simulink model "w31_v6"  (Simulink 7.9)
settings: Solver=FixedStepDiscrete  StartTime=0.0  StopTime=inf  FixedStep=0.01  RelTol=1e-3
undefined symbols (not defined in the file): DiscIntNeverNeededParam, magnitude
libraries: canmsglib x24, cansrvlib x22, simulink x12, iohwablib x5, legionoslib x3, ccpsrvlib x2, memsrvlib x1, tgttoollib x1, udssrvlib x1, wdgmlib x1
(part 4 of 5)

== system w31_v6/Logic_And_Algorithm/iECU_mode_with_control/Power_calculation/Subsystem ==
  0-1 : Saturate  UpperLimit=1  LowerLimit=0  OutDataTypeStr=uint8
  Constant : Constant  Value=0  OutDataTypeStr=uint8
  Constant1 : Constant  OutDataTypeStr=uint8
  Constant2 : Constant  Value=2  OutDataTypeStr=uint8
  Constant3 : Constant  OutDataTypeStr=uint8
  Constant4 : Constant  Value=0  OutDataTypeStr=uint8
  Constant5 : Constant  OutDataTypeStr=uint8
  Constant6 : Constant  Value=0  OutDataTypeStr=uint8
  Gain : Gain  ParamDataTypeStr=uint8
  Gain1 : Gain  ParamDataTypeStr=uint8
  Multiport Switch : MultiPortSwitch  DataPortOrder=Specify indices  DataPortIndices={0,2,1}  zeroidx=off
  Multiport Switch1 : MultiPortSwitch  DataPortOrder=Specify indices  DataPortIndices={0,1}  zeroidx=off
  Multiport Switch2 : MultiPortSwitch  DataPortOrder=Specify indices  DataPortIndices={0,1}  zeroidx=off
  Rotation_to_FL_Motor : Outport
  Rotation_to_FR_Motor : Outport  Port=2
  Rotation_to_RL_Motor : Outport  Port=3
  Rotation_to_RR_Motor : Outport  Port=4
  tag scope: iECU_GearRequestAfterCal=global
  wires:
  Multiport Switch/1 -> 0-1/1, [iECU_GearRequestAfterCal]  "Rotation_to_RL_Motor"
  Constant/1 -> Multiport Switch/2
  Constant1/1 -> Multiport Switch/3
  Constant2/1 -> Multiport Switch/4
  0-1/1 -> Gain/1, Multiport Switch1/1, Gain1/1, Multiport Switch2/1
  [iECU_GearReq] -> Multiport Switch/1
  Constant3/1 -> Multiport Switch1/2
  Constant4/1 -> Multiport Switch1/3
  Constant5/1 -> Multiport Switch2/2
  Constant6/1 -> Multiport Switch2/3
  Gain/1 -> Rotation_to_FL_Motor/1  "Rotation_to_FL_Motor"
  Multiport Switch1/1 -> Rotation_to_FR_Motor/1  "Rotation_to_FR_Motor"
  Gain1/1 -> Rotation_to_RL_Motor/1  "Rotation_to_RL_Motor"
  Multiport Switch2/1 -> Rotation_to_RR_Motor/1  "Rotation_to_RR_Motor"

== system w31_v6/Logic_And_Algorithm/iECU_mode_with_control/Signal_Input/Emg_No_Msg ==
  note: 急停或信号丢失
  No_iECU_CAN_Msg_Or_Emg_Button : Inport
  Bus Selector3 : BusSelector  OutputSignals=No_iECU_CAN_Msg_Or_Emg_Button
  tag scope: No_iECU_CAN_Msg_Or_Emg_Button=global
  wires:
  Bus Selector3/1 -> [No_iECU_CAN_Msg_Or_Emg_Button]  "<No_iECU_CAN_Msg_Or_Emg_Button>"
  No_iECU_CAN_Msg_Or_Emg_Button/1 -> Bus Selector3/1

== system w31_v6/Logic_And_Algorithm/iECU_mode_with_control/Signal_Input/Hardware_Signal_Goto ==
  Chassis_Receive_input : Inport
  Bus Selector3 : BusSelector  OutputSignals=FL_Motor_Receive.FL_RPM_Feedback,FR_Motor_Receive.FR_RPM_Feedback,RL_Motor_Receive.RL_RPM_Feedback,RR_Motor_Receive.RR_RPM_Feedback
  tag scope: iECU_FL_RPM_Feedback=global, iECU_FR_RPM_Feedback=global, iECU_RL_RPM_Feedback=global, iECU_RR_RPM_Feedback=global
  wires:
  Bus Selector3/3 -> [iECU_RL_RPM_Feedback]  "<RL_RPM_Feedback>"
  Bus Selector3/2 -> [iECU_FR_RPM_Feedback]  "<FR_RPM_Feedback>"
  Bus Selector3/1 -> [iECU_FL_RPM_Feedback]  "<FL_RPM_Feedback>"
  Chassis_Receive_input/1 -> Bus Selector3/1
  Bus Selector3/4 -> [iECU_RR_RPM_Feedback]  "<RR_RPM_Feedback>"

== system w31_v6/Logic_And_Algorithm/iECU_mode_with_control/Signal_Input/Remote_Signal_Goto ==
  Remote_CAN_input : Inport
  Bus Selector3 : BusSelector  OutputSignals=Remote_Analog.Remote_Brake_Pressure_Required
  tag scope: iECU_RemoteBrakePressure=global
  wires:
  Remote_CAN_input/1 -> Bus Selector3/1
  Bus Selector3/1 -> [iECU_RemoteBrakePressure]  "<Remote_Brake_Pressure_Required>"

== system w31_v6/Logic_And_Algorithm/iECU_mode_with_control/Signal_Input/iECU_Signal_Goto ==
  iECU_CAN_input : Inport
  -30~+30 : Saturate  UpperLimit=30  LowerLimit=-30  OutDataTypeStr=Inherit: Inherit via back propagation
  -30~30 : Saturate  UpperLimit=30  LowerLimit=-30  OutDataTypeStr=Inherit: Inherit via back propagation
  Bus Selector3 : BusSelector  OutputSignals=iECU_Speed_Required,iECU_FTire_Angle_Rrquired,iECU_RTire_Angle_Rrquired,iECU_Brake_Pressure_Required,iECU_EPB_Req,iECU_Control_Flag,iECU_Gear_Required,iECU_FTire_Angle_Rrquired,iECU_RTire_Angle_Rrquired,iECU_Status
  tag scope: iECU_BrakePressureReq=global, iECU_Control_Flag=global, iECU_EPB_Req=global, iECU_FTire_Angle_Rrquired=global, iECU_GearReq=global, iECU_RTire_Angle_Rrquired=global, iECU_SpeedLimReq=global, iECU_SpeedReq=global, iECU_Status=global, iECU_SteerModeReq=global
  wires:
  iECU_CAN_input/1 -> Bus Selector3/1
  Bus Selector3/1 -> [iECU_SpeedReq]  "<iECU_Speed_Required>"
  Bus Selector3/2 -> -30~+30/1  "<iECU_FTire_Angle_Rrquired>"
  -30~+30/1 -> [iECU_FTire_Angle_Rrquired]
  Bus Selector3/3 -> -30~30/1  "<iECU_RTire_Angle_Rrquired>"
  -30~30/1 -> [iECU_RTire_Angle_Rrquired]
  Bus Selector3/4 -> [iECU_BrakePressureReq]  "<iECU_Brake_Pressure_Required>"
  Bus Selector3/5 -> [iECU_EPB_Req]  "<iECU_EPB_Req>"
  Bus Selector3/6 -> [iECU_Control_Flag]  "<iECU_Control_Flag>"
  Bus Selector3/7 -> [iECU_GearReq]  "<iECU_Gear_Required>"
  Bus Selector3/8 -> [iECU_SpeedLimReq]  "<iECU_FTire_Angle_Rrquired>"
  Bus Selector3/9 -> [iECU_SteerModeReq]  "<iECU_RTire_Angle_Rrquired>"
  Bus Selector3/10 -> [iECU_Status]  "<iECU_Status>"

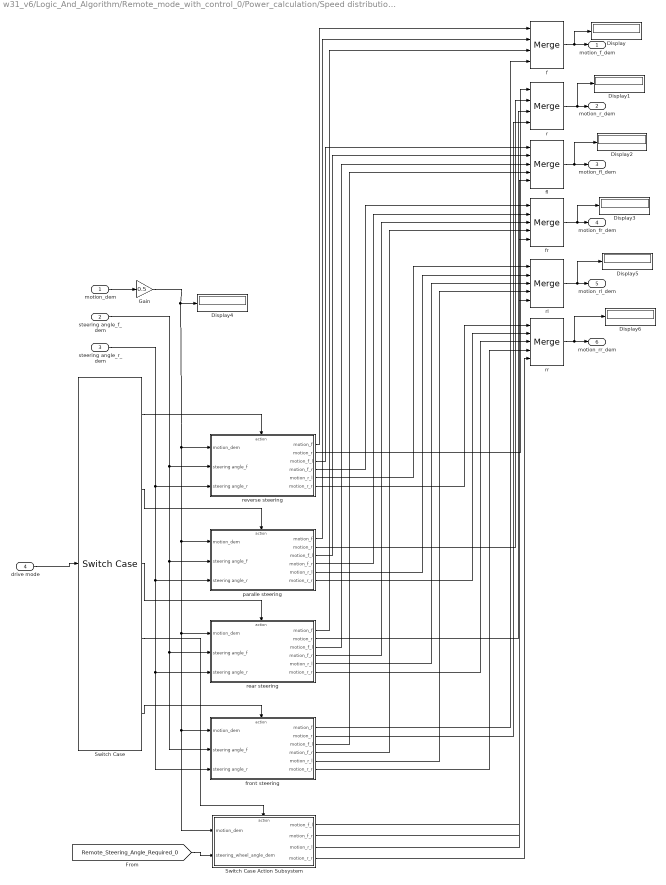
== system w31_v6/Logic_And_Algorithm/Remote_mode_with_control_0/Power_calculation/Speed distribution strategy/motion distribution1 ==
  motion_dem : Inport
  steering angle_f_dem : Inport  Port=2
  steering angle_r_dem : Inport  Port=3
  drive mode : Inport  Port=4
  Display{,1..6} (7 alike) : Display
  Gain : Gain  Gain=0.5
  Switch Case : SwitchCase  CaseConditions={3,0,2,4}
  Switch Case Action Subsystem : Subsystem  TreatAsAtomicUnit=on
  f : Merge  Inputs=4
  fl : Merge  Inputs=5
  fr : Merge  Inputs=5
  front steering : Subsystem  TreatAsAtomicUnit=on
  paralle steering : Subsystem  TreatAsAtomicUnit=on
  r : Merge  Inputs=4
  rear steering : Subsystem  TreatAsAtomicUnit=on
  reverse steering : Subsystem  TreatAsAtomicUnit=on
  rl : Merge  Inputs=5
  rr : Merge  Inputs=5
  motion_f_dem : Outport
  motion_r_dem : Outport  Port=2
  motion_fl_dem : Outport  Port=3
  motion_fr_dem : Outport  Port=4
  motion_rl_dem : Outport  Port=5
  motion_rr_dem : Outport  Port=6
  wires:
  drive mode/1 -> Switch Case/1
  Switch Case/1 -> reverse steering/Action
  Switch Case/2 -> paralle steering/Action
  Switch Case/5 -> front steering/Action
  Switch Case/3 -> rear steering/Action
  reverse steering/3(motion_f_l) -> fl/1
  reverse steering/4(motion_f_r) -> fr/1
  reverse steering/6(motion_r_r) -> rr/1
  paralle steering/3(motion_f_l) -> fl/2
  rear steering/3(motion_f_l) -> fl/3
  front steering/3(motion_f_l) -> fl/4
  paralle steering/4(motion_f_r) -> fr/2
  rear steering/4(motion_f_r) -> fr/3
  front steering/4(motion_f_r) -> fr/4
  reverse steering/5(motion_r_l) -> rl/1
  paralle steering/5(motion_r_l) -> rl/2
  rear steering/5(motion_r_l) -> rl/3
  front steering/5(motion_r_l) -> rl/4
  paralle steering/6(motion_r_r) -> rr/2
  rear steering/6(motion_r_r) -> rr/3
  front steering/6(motion_r_r) -> rr/4
  rr/1 -> motion_rr_dem/1, Display6/1
  rl/1 -> motion_rl_dem/1, Display5/1
  fr/1 -> motion_fr_dem/1, Display3/1
  fl/1 -> motion_fl_dem/1, Display2/1
  f/1 -> motion_f_dem/1, Display/1
  r/1 -> motion_r_dem/1, Display1/1
  reverse steering/1(motion_f) -> f/1
  paralle steering/1(motion_f) -> f/2
  rear steering/1(motion_f) -> f/3
  front steering/1(motion_f) -> f/4
  reverse steering/2(motion_r) -> r/1
  paralle steering/2(motion_r) -> r/2
  rear steering/2(motion_r) -> r/3
  front steering/2(motion_r) -> r/4
  motion_dem/1 -> Gain/1
  steering angle_f_dem/1 -> paralle steering/2(steering angle_f), rear steering/2(steering angle_f), front steering/2(steering angle_f), reverse steering/2(steering angle_f)
  steering angle_r_dem/1 -> reverse steering/3(steering angle_r), rear steering/3(steering angle_r), front steering/3(steering angle_r), paralle steering/3(steering angle_r)
  Switch Case/4 -> Switch Case Action Subsystem/Action
  Switch Case Action Subsystem/1(motion_f_l) -> fl/5
  Switch Case Action Subsystem/2(motion_f_r) -> fr/5
  Switch Case Action Subsystem/3(motion_r_l) -> rl/5
  Switch Case Action Subsystem/4(motion_r_r) -> rr/5
  [Remote_Steering_Angle_Required_0] -> Switch Case Action Subsystem/2(steering_wheel_angle_dem)
  Gain/1 -> reverse steering/1(motion_dem), rear steering/1(motion_dem), front steering/1(motion_dem), Switch Case Action Subsystem/1(motion_dem), paralle steering/1(motion_dem), Display4/1

== system w31_v6/Logic_And_Algorithm/Remote_mode_with_control_0/Steering_calculation/Angle_Cal/F_Steer_mode ==
  Remote_steering : Inport
  Action Port : ActionPort  ActionType=default
  Gain : Gain  Gain=1.2
  Gain1 : Gain  Gain=0
  F_Steering_Angle : Outport
  R_Steering_Angle : Outport  Port=2
  wires:
  Remote_steering/1 -> Gain/1, Gain1/1  "Remote_Steering_Request"
  Gain/1 -> F_Steering_Angle/1  "F_Steering_Angle"
  Gain1/1 -> R_Steering_Angle/1  "R_Steering_Angle"

== system w31_v6/Logic_And_Algorithm/Remote_mode_with_control_0/Steering_calculation/Angle_Cal/Parallel_Steer_mode ==
  Remote_steering : Inport
  Action Port : ActionPort  ActionType=case
  Gain1 : Gain  Gain=1.2
  Tire2EPS : Gain  Gain=1.2
  F_Steering_Angle : Outport
  R_Steering_Angle : Outport  Port=2
  wires:
  Remote_steering/1 -> Tire2EPS/1, Gain1/1  "Remote_Steering_Request"
  Tire2EPS/1 -> F_Steering_Angle/1  "F_Steering_Angle"
  Gain1/1 -> R_Steering_Angle/1  "R_Steering_Angle"

== system w31_v6/Logic_And_Algorithm/Remote_mode_with_control_0/Steering_calculation/Angle_Cal/R_Steer_mode ==
  Remote_steering : Inport
  Action Port : ActionPort  ActionType=case
  Gain : Gain  Gain=0
  Gain1 : Gain  Gain=1.2
  F_Steering_Angle : Outport
  R_Steering_Angle : Outport  Port=2
  wires:
  Remote_steering/1 -> Gain/1, Gain1/1  "Remote_Steering_Request"
  Gain/1 -> F_Steering_Angle/1  "F_Steering_Angle"
  Gain1/1 -> R_Steering_Angle/1  "R_Steering_Angle"

== system w31_v6/Logic_And_Algorithm/Remote_mode_with_control_0/Steering_calculation/Angle_Cal/Reverse_Steer_mode ==
  Remote_steering : Inport
  Action Port : ActionPort  ActionType=case
  Gain : Gain  Gain=1.2
  Gain1 : Gain  Gain=-1.2
  F_Steering_Angle : Outport
  R_Steering_Angle : Outport  Port=2
  wires:
  Remote_steering/1 -> Gain/1, Gain1/1  "Remote_Steering_Request"
  Gain/1 -> F_Steering_Angle/1  "F_Steering_Angle"
  Gain1/1 -> R_Steering_Angle/1  "R_Steering_Angle"

== system w31_v6/Logic_And_Algorithm/Remote_mode_with_control_0/Steering_calculation/Angle_Cal/Steer_Model_Judge ==
  Data Type Conversion : DataTypeConversion  OutDataTypeStr=double
  Data Type Conversion1 : DataTypeConversion  OutDataTypeStr=double
  Data Type Conversion2 : DataTypeConversion  OutDataTypeStr=uint8
  MATLAB Function : MATLAB Function  TreatAsAtomicUnit=on
  Steering_mode : Outport
  tag scope: steering_mode_0=global
  wires:
  MATLAB Function/1(mode) -> Data Type Conversion2/1
  Data Type Conversion/1 -> MATLAB Function/1(steer_gear)
  Data Type Conversion1/1 -> MATLAB Function/2(D_button)
  Data Type Conversion2/1 -> Steering_mode/1, [steering_mode_0]
  [Remote_Steering_Mode_Switch1_0] -> Data Type Conversion/1
  [Remote_Steering_Mode_Switch2_0] -> Data Type Conversion1/1

== system w31_v6/Logic_And_Algorithm/Remote_mode_with_control_0/Steering_calculation/Angle_Cal/turn_in_place ==
  Remote_steering : Inport
  Action Port : ActionPort  ActionType=case
  Gain : Gain  Gain=0
  Gain1 : Gain  Gain=0
  Gain2 : Gain
  F_Steering_Angle : Outport
  R_Steering_Angle : Outport  Port=2
  wires:
  Remote_steering/1 -> Gain2/1  "Remote_Steering_Request"
  Gain/1 -> F_Steering_Angle/1  "F_Steering_Angle"
  Gain1/1 -> R_Steering_Angle/1  "R_Steering_Angle"
  Gain2/1 -> Gain/1, Gain1/1

== system w31_v6/Logic_And_Algorithm/Remote_mode_with_control_2/Steering_calculation/Angle_Cal/F_Steer_mode ==
  Remote_steering : Inport
  Action Port : ActionPort  ActionType=default
  Gain : Gain
  Gain1 : Gain  Gain=0
  F_Steering_Angle : Outport
  R_Steering_Angle : Outport  Port=2
  wires:
  Gain1/1 -> R_Steering_Angle/1  "R_Steering_Angle"
  Gain/1 -> F_Steering_Angle/1  "F_Steering_Angle"
  Remote_steering/1 -> Gain1/1, Gain/1  "Remote_Steering_Request"

== system w31_v6/Logic_And_Algorithm/Remote_mode_with_control_2/Steering_calculation/Angle_Cal/Parallel_Steer_mode ==
  Remote_steering : Inport
  Action Port : ActionPort  ActionType=case
  Gain1 : Gain
  Tire2EPS : Gain
  F_Steering_Angle : Outport
  R_Steering_Angle : Outport  Port=2
  wires:
  Gain1/1 -> R_Steering_Angle/1  "R_Steering_Angle"
  Tire2EPS/1 -> F_Steering_Angle/1  "F_Steering_Angle"
  Remote_steering/1 -> Gain1/1, Tire2EPS/1  "Remote_Steering_Request"

== system w31_v6/Logic_And_Algorithm/Remote_mode_with_control_2/Steering_calculation/Angle_Cal/R_Steer_mode ==
  Remote_steering : Inport
  Action Port : ActionPort  ActionType=case
  Gain : Gain  Gain=0
  Gain1 : Gain
  F_Steering_Angle : Outport
  R_Steering_Angle : Outport  Port=2
  wires:
  Gain1/1 -> R_Steering_Angle/1  "R_Steering_Angle"
  Gain/1 -> F_Steering_Angle/1  "F_Steering_Angle"
  Remote_steering/1 -> Gain1/1, Gain/1  "Remote_Steering_Request"

== system w31_v6/Logic_And_Algorithm/Remote_mode_with_control_2/Steering_calculation/Angle_Cal/Reverse_Steer_mode ==
  Remote_steering : Inport
  Action Port : ActionPort  ActionType=case
  Gain : Gain
  Gain1 : Gain  Gain=-1
  F_Steering_Angle : Outport
  R_Steering_Angle : Outport  Port=2
  wires:
  Gain1/1 -> R_Steering_Angle/1  "R_Steering_Angle"
  Gain/1 -> F_Steering_Angle/1  "F_Steering_Angle"
  Remote_steering/1 -> Gain1/1, Gain/1  "Remote_Steering_Request"

== system w31_v6/Logic_And_Algorithm/Remote_mode_with_control_2/Steering_calculation/Angle_Cal/Steer_Model_Judge ==
  Data Type Conversion : DataTypeConversion  OutDataTypeStr=double
  Data Type Conversion1 : DataTypeConversion  OutDataTypeStr=double
  Data Type Conversion2 : DataTypeConversion  OutDataTypeStr=uint8
  MATLAB Function : MATLAB Function  TreatAsAtomicUnit=on
  Steering_model : Outport
  tag scope: steering_drive_mode2=global
  wires:
  [Remote_Steering_Mode_Switch2_2] -> Data Type Conversion1/1
  [Remote_Steering_Mode_Switch1_2] -> Data Type Conversion/1
  Data Type Conversion2/1 -> Steering_model/1, [steering_drive_mode2]
  Data Type Conversion1/1 -> MATLAB Function/2(D_button)
  Data Type Conversion/1 -> MATLAB Function/1(steer_gear)
  MATLAB Function/1(mode) -> Data Type Conversion2/1

== system w31_v6/Logic_And_Algorithm/Remote_mode_with_control_2/Steering_calculation/Angle_Cal/turn_in_place ==
  Remote_steering : Inport
  Action Port : ActionPort  ActionType=case
  Gain : Gain  Gain=0
  Gain1 : Gain  Gain=0
  Gain2 : Gain
  F_Steering_Angle : Outport
  R_Steering_Angle : Outport  Port=2
  wires:
  Remote_steering/1 -> Gain2/1  "Remote_Steering_Request"
  Gain/1 -> F_Steering_Angle/1  "F_Steering_Angle"
  Gain1/1 -> R_Steering_Angle/1  "R_Steering_Angle"
  Gain2/1 -> Gain/1, Gain1/1

== system w31_v6/Logic_And_Algorithm/iECU_mode_with_control/Power_calculation/PID_Controller/FL_PI_Cal2 ==
  FL_Motor_Error : Inport
  Constant : Constant
  Constant1 : Constant  Value=1.5
  Constant3 : Constant  Value=0
  Constant4 : Constant  Value=0  SampleTime=-1
  Constant5 : Constant  SampleTime=-1
  PI : Subsystem
  Switch : Switch  Criteria=u2 > Threshold
  Switch1 : Switch  Criteria=u2 > Threshold
  Torque_to_FL_Motor : Outport
  wires:
  Constant5/1 -> Switch1/1
  Constant4/1 -> Switch1/3
  [iECU_PID_Reset] -> Switch1/2
  Switch/1 -> Torque_to_FL_Motor/1
  PI/1(PI_闭环计算扭矩) -> Switch/3
  FL_Motor_Error/1 -> PI/1(Error)
  Constant3/1 -> Switch/1
  [iECU_PID_Reset] -> Switch/2
  Constant1/1 -> PI/4(Pgain)
  Constant/1 -> PI/3(Igain)
  Switch1/1 -> PI/2(PID_Reset)

== system w31_v6/Logic_And_Algorithm/iECU_mode_with_control/Power_calculation/PID_Controller/FR_PI_Cal1 ==
  FR_Motor_Error : Inport
  Constant : Constant
  Constant1 : Constant  Value=1.5
  Constant3 : Constant  Value=0
  Constant4 : Constant  Value=0  SampleTime=-1
  Constant5 : Constant  SampleTime=-1
  PI : Subsystem
  Switch : Switch  Criteria=u2 > Threshold
  Switch1 : Switch  Criteria=u2 > Threshold
  Torque_to_FR_Motor : Outport
  wires:
  Switch1/1 -> PI/2(PID_Reset)
  Constant/1 -> PI/3(Igain)
  Constant1/1 -> PI/4(Pgain)
  [iECU_PID_Reset] -> Switch/2
  Constant3/1 -> Switch/1
  FR_Motor_Error/1 -> PI/1(Error)
  PI/1(PI_闭环计算扭矩) -> Switch/3
  Switch/1 -> Torque_to_FR_Motor/1
  [iECU_PID_Reset] -> Switch1/2
  Constant4/1 -> Switch1/3
  Constant5/1 -> Switch1/1

== system w31_v6/Logic_And_Algorithm/iECU_mode_with_control/Power_calculation/PID_Controller/RL_PI_Cal ==
  RL_Motor_Error : Inport
  Constant : Constant
  Constant1 : Constant  Value=1.5
  Constant2 : Constant  Value=0  SampleTime=-1
  Constant3 : Constant  Value=0
  Constant4 : Constant  SampleTime=-1
  PI : Subsystem
  Switch : Switch  Criteria=u2 > Threshold
  Switch1 : Switch  Criteria=u2 > Threshold
  Torque_to_RL_Motor : Outport
  wires:
  Constant/1 -> PI/3(Igain)
  Constant1/1 -> PI/4(Pgain)
  [iECU_PID_Reset] -> Switch/2
  Constant3/1 -> Switch/1
  PI/1(PI_闭环计算扭矩) -> Switch/3
  Switch/1 -> Torque_to_RL_Motor/1
  RL_Motor_Error/1 -> PI/1(Error)
  [iECU_PID_Reset] -> Switch1/2
  Constant2/1 -> Switch1/3
  Constant4/1 -> Switch1/1
  Switch1/1 -> PI/2(PID_Reset)

== system w31_v6/Logic_And_Algorithm/iECU_mode_with_control/Power_calculation/PID_Controller/RR_PI_Cal ==
  RR_Motor_Error : Inport
  Constant : Constant
  Constant1 : Constant  Value=1.5
  Constant3 : Constant  Value=0
  Constant4 : Constant  Value=0  SampleTime=-1
  Constant5 : Constant  SampleTime=-1
  PI : Subsystem
  Switch : Switch  Criteria=u2 > Threshold
  Switch1 : Switch  Criteria=u2 > Threshold
  Torque_to_RR_Motor : Outport
  wires:
  Switch1/1 -> PI/2(PID_Reset)
  Constant/1 -> PI/3(Igain)
  Constant1/1 -> PI/4(Pgain)
  [iECU_PID_Reset] -> Switch/2
  Constant3/1 -> Switch/1
  RR_Motor_Error/1 -> PI/1(Error)
  PI/1(PI_闭环计算扭矩) -> Switch/3
  Switch/1 -> Torque_to_RR_Motor/1
  [iECU_PID_Reset] -> Switch1/2
  Constant4/1 -> Switch1/3
  Constant5/1 -> Switch1/1

== system w31_v6/Logic_And_Algorithm/Remote_mode_with_control_0/Power_calculation/Speed distribution strategy/motion distribution1/Switch Case Action Subsystem ==
  note: 做一个原地转向的限制，轮速不能高于50RPM
  motion_dem : Inport
  steering_wheel_angle_dem : Inport  Port=2
  Action Port : ActionPort  ActionType=case
  MATLAB Function : MATLAB Function  TreatAsAtomicUnit=on
  Product{,1..3} (4 alike) : Product  RndMeth=Zero
  Saturation : Saturate  UpperLimit=50  LowerLimit=-50
  motion_f_l : Outport
  motion_f_r : Outport  Port=2
  motion_r_l : Outport  Port=3
  motion_r_r : Outport  Port=4
  wires:
  steering_wheel_angle_dem/1 -> MATLAB Function/1(steering_wheel_angle_dem)
  motion_dem/1 -> Saturation/1
  MATLAB Function/1(gain1) -> Product/2
  MATLAB Function/2(gain2) -> Product1/2
  MATLAB Function/3(gain3) -> Product2/2
  MATLAB Function/4(gain4) -> Product3/2
  Product/1 -> motion_f_l/1
  Product1/1 -> motion_f_r/1
  Product2/1 -> motion_r_l/1
  Product3/1 -> motion_r_r/1
  Saturation/1 -> Product/1, Product1/1, Product3/1, Product2/1

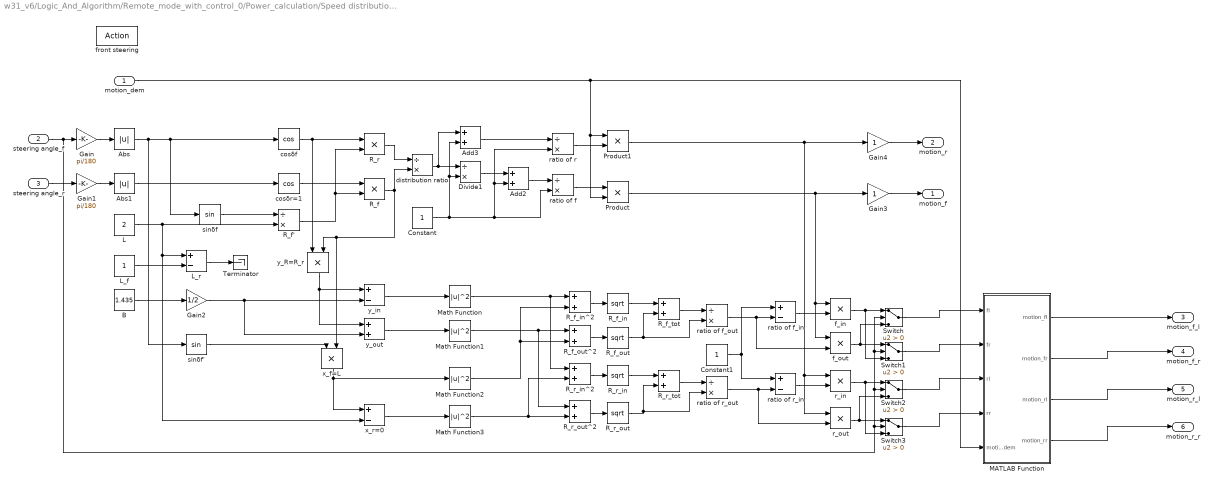
== system w31_v6/Logic_And_Algorithm/Remote_mode_with_control_0/Power_calculation/Speed distribution strategy/motion distribution1/front steering ==
  motion_dem : Inport
  steering angle_f : Inport  Port=2
  steering angle_r : Inport  Port=3
  front steering : ActionPort  ActionType=default
  Abs : Abs
  Abs1 : Abs
  Add2 : Sum
  Add3 : Sum
  B : Constant  Value=1.435
  Constant : Constant
  Constant1 : Constant
  Divide1 : Product  Inputs=/*
  Gain : Gain  Gain=pi/180
  Gain1 : Gain  Gain=pi/180
  Gain2 : Gain  Gain=1/2
  Gain3 : Gain
  Gain4 : Gain
  L : Constant  Value=2
  L_f : Constant
  L_r : Sum  Inputs=+-
  MATLAB Function : MATLAB Function  TreatAsAtomicUnit=on
  Math Function{,1..3} (4 alike) : Math  Operator=magnitude^2  SaturateOnIntegerOverflow=on
  Product : Product
  Product1 : Product
  R_f : Product
  R_f' : Product  Inputs=/*
  R_f_in : Sqrt  SaturateOnIntegerOverflow=on
  R_f_in^2 : Sum
  R_f_out : Sqrt  SaturateOnIntegerOverflow=on
  R_f_out^2 : Sum
  R_f_tot : Sum
  R_r : Product
  R_r_in : Sqrt  SaturateOnIntegerOverflow=on
  R_r_in^2 : Sum
  R_r_out : Sqrt  SaturateOnIntegerOverflow=on
  R_r_out^2 : Sum
  R_r_tot : Sum
  Switch{,1..3} (4 alike) : Switch  Criteria=u2 > Threshold
  Terminator : Terminator
  cosδf : Trigonometry  Operator=cos
  cosδr=1 : Trigonometry  Operator=cos
  distribution ratio : Product  Inputs=/*
  f_in : Product
  f_out : Product
  r_in : Product
  r_out : Product
  ratio of f : Product  Inputs=/*
  ratio of f_in : Sum  Inputs=+-
  ratio of f_out : Product  Inputs=/*
  ratio of r : Product  Inputs=/*
  ratio of r_in : Sum  Inputs=+-
  ratio of r_out : Product  Inputs=/*
  sinδf : Trigonometry
  sinδf' : Trigonometry
  x_f=L : Product
  x_r=0 : Sum  Inputs=+-
  y_R=R_r : Product
  y_in : Sum  Inputs=+-
  y_out : Sum
  motion_f : Outport
  motion_r : Outport  Port=2
  motion_f_l : Outport  Port=3
  motion_f_r : Outport  Port=4
  motion_r_l : Outport  Port=5
  motion_r_r : Outport  Port=6
  wires:
  r_out/1 -> Switch3/1, Switch2/3
  f_out/1 -> Switch1/1, Switch/3
  r_in/1 -> Switch3/3, Switch2/1
  f_in/1 -> Switch/1, Switch1/3
  ratio of f_in/1 -> f_in/2
  ratio of r_in/1 -> r_in/2
  Constant1/1 -> ratio of r_in/1, ratio of f_in/1
  ratio of r_out/1 -> ratio of r_in/2, r_out/2
  ratio of f_out/1 -> ratio of f_in/2, f_out/2
  R_r_tot/1 -> ratio of r_out/1
  R_f_tot/1 -> ratio of f_out/1
  R_r_out/1 -> R_r_tot/2, ratio of r_out/2
  R_r_in/1 -> R_r_tot/1
  R_f_out/1 -> R_f_tot/2, ratio of f_out/2
  R_f_in/1 -> R_f_tot/1
  R_r_out^2/1 -> R_r_out/1
  R_f_out^2/1 -> R_f_out/1
  R_r_in^2/1 -> R_r_in/1
  R_f_in^2/1 -> R_f_in/1
  Math Function3/1 -> R_r_in^2/2, R_r_out^2/2
  Math Function1/1 -> R_f_out^2/1, R_r_out^2/1
  Math Function2/1 -> R_f_in^2/2, R_f_out^2/2
  Math Function/1 -> R_f_in^2/1, R_r_in^2/1
  x_r=0/1 -> Math Function3/1
  y_out/1 -> Math Function1/1
  y_in/1 -> Math Function/1
  x_f=L/1 -> Math Function2/1, x_r=0/1
  L_r/1 -> Terminator/1
  sinδf'/1 -> x_f=L/1
  Gain2/1 -> y_in/2, y_out/2
  y_R=R_r/1 -> y_in/1, y_out/1
  B/1 -> Gain2/1
  Gain1/1 -> Abs1/1
  steering angle_r/1 -> Gain1/1
  Gain/1 -> Abs/1
  steering angle_f/1 -> Gain/1, Switch2/2, Switch/2, Switch1/2, Switch3/2
  Product/1 -> f_out/1, f_in/1, Gain3/1
  Product1/1 -> r_in/1, r_out/1, Gain4/1
  ratio of f/1 -> Product/1
  ratio of r/1 -> Product1/2
  motion_dem/1 -> Product1/1, Product/2, MATLAB Function/5(motion_dem)
  Add3/1 -> ratio of r/1
  Add2/1 -> ratio of f/1
  Divide1/1 -> Add2/1
  Constant/1 -> Divide1/2, Add3/2, Add2/2, ratio of r/2, ratio of f/2
  distribution ratio/1 -> Divide1/1, Add3/1
  R_r/1 -> distribution ratio/1
  R_f/1 -> x_f=L/2, y_R=R_r/2, distribution ratio/2
  R_f'/1 -> R_f/2, R_r/2
  cosδr=1/1 -> R_f/1
  cosδf/1 -> y_R=R_r/1, R_r/1
  sinδf/1 -> R_f'/1
  Abs1/1 -> cosδr=1/1
  Abs/1 -> sinδf/1, cosδf/1, sinδf'/1
  L_f/1 -> L_r/2
  L/1 -> x_r=0/2, L_r/1, R_f'/2
  Gain3/1 -> motion_f/1
  Gain4/1 -> motion_r/1
  Switch/1 -> MATLAB Function/1(fl)
  Switch1/1 -> MATLAB Function/2(fr)
  Switch2/1 -> MATLAB Function/3(rl)
  Switch3/1 -> MATLAB Function/4(rr)
  MATLAB Function/1(motion_fl) -> motion_f_l/1
  MATLAB Function/2(motion_fr) -> motion_f_r/1
  MATLAB Function/3(motion_rl) -> motion_r_l/1
  MATLAB Function/4(motion_rr) -> motion_r_r/1

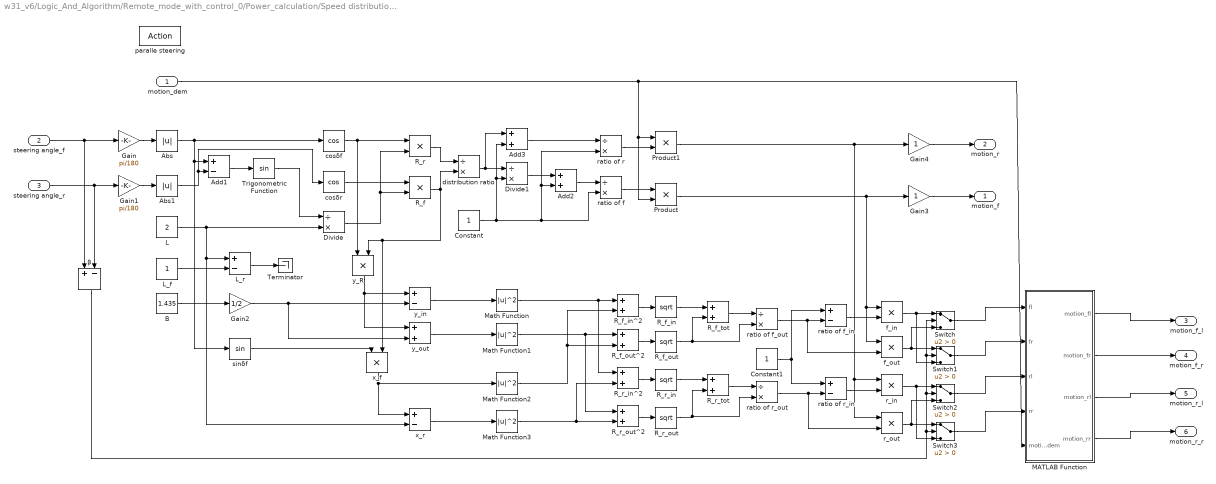
== system w31_v6/Logic_And_Algorithm/Remote_mode_with_control_0/Power_calculation/Speed distribution strategy/motion distribution1/paralle steering ==
  motion_dem : Inport
  steering angle_f : Inport  Port=2
  steering angle_r : Inport  Port=3
  paralle steering : ActionPort  ActionType=case
  Abs : Abs
  Abs1 : Abs
  Add1 : Sum  Inputs=+-
  Add2 : Sum
  Add3 : Sum
  B : Constant  Value=1.435
  Constant : Constant
  Constant1 : Constant
  Divide : Product  Inputs=/*
  Divide1 : Product  Inputs=/*
  Gain : Gain  Gain=pi/180
  Gain1 : Gain  Gain=pi/180
  Gain2 : Gain  Gain=1/2
  Gain3 : Gain
  Gain4 : Gain
  L : Constant  Value=2
  L_f : Constant
  L_r : Sum  Inputs=+-
  MATLAB Function : MATLAB Function  TreatAsAtomicUnit=on
  Math Function{,1..3} (4 alike) : Math  Operator=magnitude^2  SaturateOnIntegerOverflow=on
  Product : Product
  Product1 : Product
  R_f : Product
  R_f_in : Sqrt  SaturateOnIntegerOverflow=on
  R_f_in^2 : Sum
  R_f_out : Sqrt  SaturateOnIntegerOverflow=on
  R_f_out^2 : Sum
  R_f_tot : Sum
  R_r : Product
  R_r_in : Sqrt  SaturateOnIntegerOverflow=on
  R_r_in^2 : Sum
  R_r_out : Sqrt  SaturateOnIntegerOverflow=on
  R_r_out^2 : Sum
  R_r_tot : Sum
  Switch{,1..3} (4 alike) : Switch  Criteria=u2 > Threshold
  Terminator : Terminator
  Trigonometric Function : Trigonometry
  cosδf : Trigonometry  Operator=cos
  cosδr : Trigonometry  Operator=cos
  distribution ratio : Product  Inputs=/*
  f_in : Product
  f_out : Product
  r_in : Product
  r_out : Product
  ratio of f : Product  Inputs=/*
  ratio of f_in : Sum  Inputs=+-
  ratio of f_out : Product  Inputs=/*
  ratio of r : Product  Inputs=/*
  ratio of r_in : Sum  Inputs=+-
  ratio of r_out : Product  Inputs=/*
  sinδf : Trigonometry
  x_f : Product
  x_r : Sum  Inputs=+-
  y_R : Product
  y_in : Sum  Inputs=+-
  y_out : Sum
  β : Sum  Inputs=+-
  motion_f : Outport
  motion_r : Outport  Port=2
  motion_f_l : Outport  Port=3
  motion_f_r : Outport  Port=4
  motion_r_l : Outport  Port=5
  motion_r_r : Outport  Port=6
  wires:
  r_out/1 -> Switch3/1, Switch2/3
  f_out/1 -> Switch1/1, Switch/3
  r_in/1 -> Switch3/3, Switch2/1
  f_in/1 -> Switch/1, Switch1/3
  ratio of f_in/1 -> f_in/2
  ratio of r_in/1 -> r_in/2
  Constant1/1 -> ratio of r_in/1, ratio of f_in/1
  ratio of r_out/1 -> ratio of r_in/2, r_out/2
  ratio of f_out/1 -> ratio of f_in/2, f_out/2
  R_r_tot/1 -> ratio of r_out/1
  R_f_tot/1 -> ratio of f_out/1
  R_r_out/1 -> R_r_tot/2, ratio of r_out/2
  R_r_in/1 -> R_r_tot/1
  R_f_out/1 -> R_f_tot/2, ratio of f_out/2
  R_f_in/1 -> R_f_tot/1
  R_r_out^2/1 -> R_r_out/1
  R_f_out^2/1 -> R_f_out/1
  R_r_in^2/1 -> R_r_in/1
  R_f_in^2/1 -> R_f_in/1
  Math Function3/1 -> R_r_in^2/2, R_r_out^2/2
  Math Function1/1 -> R_f_out^2/1, R_r_out^2/1
  Math Function2/1 -> R_f_in^2/2, R_f_out^2/2
  Math Function/1 -> R_f_in^2/1, R_r_in^2/1
  x_r/1 -> Math Function3/1
  y_out/1 -> Math Function1/1
  y_in/1 -> Math Function/1
  x_f/1 -> Math Function2/1, x_r/1
  L_r/1 -> Terminator/1
  sinδf/1 -> x_f/1
  Gain2/1 -> y_in/2, y_out/2
  y_R/1 -> y_in/1, y_out/1
  B/1 -> Gain2/1
  Gain1/1 -> Abs1/1
  steering angle_r/1 -> Gain1/1, β/2
  Gain/1 -> Abs/1
  β/1 -> Switch2/2, Switch/2, Switch1/2, Switch3/2
  Product/1 -> f_out/1, f_in/1, Gain3/1
  Product1/1 -> r_in/1, r_out/1, Gain4/1
  ratio of f/1 -> Product/1
  ratio of r/1 -> Product1/2
  motion_dem/1 -> Product1/1, Product/2, MATLAB Function/5(motion_dem)
  Add3/1 -> ratio of r/1
  Add2/1 -> ratio of f/1
  Divide1/1 -> Add2/1
  Constant/1 -> Divide1/2, Add3/2, Add2/2, ratio of r/2, ratio of f/2
  distribution ratio/1 -> Divide1/1, Add3/1
  R_r/1 -> distribution ratio/1
  R_f/1 -> distribution ratio/2, x_f/2, y_R/2
  Divide/1 -> R_r/2, R_f/2
  cosδr/1 -> R_f/1
  cosδf/1 -> y_R/1, R_r/1
  Trigonometric Function/1 -> Divide/1
  Add1/1 -> Trigonometric Function/1
  Abs1/1 -> Add1/2, cosδr/1
  Abs/1 -> cosδf/1, Add1/1, sinδf/1
  L_f/1 -> L_r/2
  L/1 -> x_r/2, L_r/1, Divide/2
  steering angle_f/1 -> β/1, Gain/1
  Gain3/1 -> motion_f/1
  Gain4/1 -> motion_r/1
  Switch/1 -> MATLAB Function/1(fl)
  Switch1/1 -> MATLAB Function/2(fr)
  Switch2/1 -> MATLAB Function/3(rl)
  Switch3/1 -> MATLAB Function/4(rr)
  MATLAB Function/1(motion_fl) -> motion_f_l/1
  MATLAB Function/2(motion_fr) -> motion_f_r/1
  MATLAB Function/3(motion_rl) -> motion_r_l/1
  MATLAB Function/4(motion_rr) -> motion_r_r/1

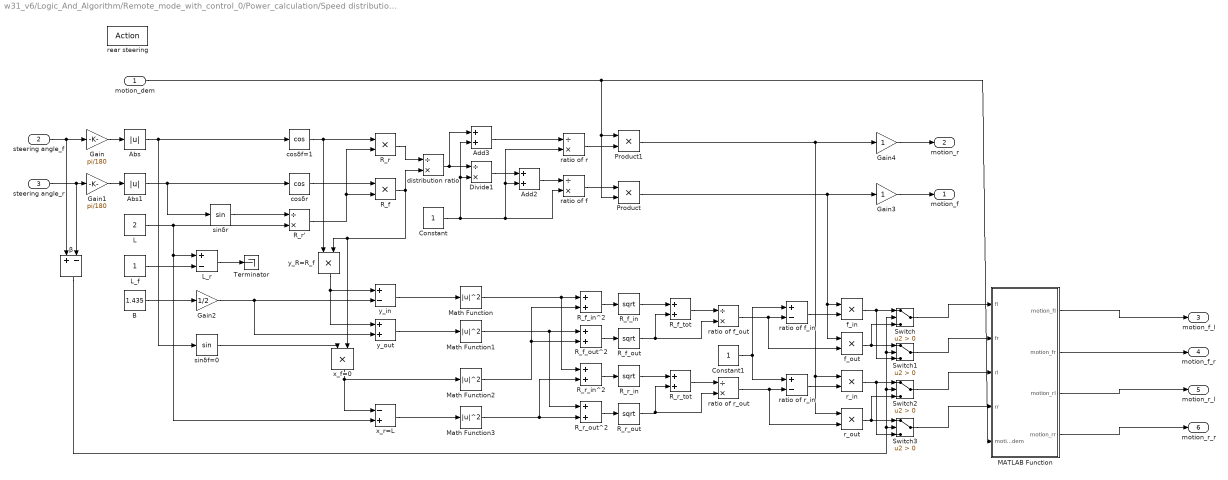
== system w31_v6/Logic_And_Algorithm/Remote_mode_with_control_0/Power_calculation/Speed distribution strategy/motion distribution1/rear steering ==
  motion_dem : Inport
  steering angle_f : Inport  Port=2
  steering angle_r : Inport  Port=3
  rear steering : ActionPort  ActionType=case
  Abs : Abs
  Abs1 : Abs
  Add2 : Sum
  Add3 : Sum
  B : Constant  Value=1.435
  Constant : Constant
  Constant1 : Constant
  Divide1 : Product  Inputs=/*
  Gain : Gain  Gain=pi/180
  Gain1 : Gain  Gain=pi/180
  Gain2 : Gain  Gain=1/2
  Gain3 : Gain
  Gain4 : Gain
  L : Constant  Value=2
  L_f : Constant
  L_r : Sum  Inputs=+-
  MATLAB Function : MATLAB Function  TreatAsAtomicUnit=on
  Math Function{,1..3} (4 alike) : Math  Operator=magnitude^2  SaturateOnIntegerOverflow=on
  Product : Product
  Product1 : Product
  R_f : Product
  R_f_in : Sqrt  SaturateOnIntegerOverflow=on
  R_f_in^2 : Sum
  R_f_out : Sqrt  SaturateOnIntegerOverflow=on
  R_f_out^2 : Sum
  R_f_tot : Sum
  R_r : Product
  R_r' : Product  Inputs=/*
  R_r_in : Sqrt  SaturateOnIntegerOverflow=on
  R_r_in^2 : Sum
  R_r_out : Sqrt  SaturateOnIntegerOverflow=on
  R_r_out^2 : Sum
  R_r_tot : Sum
  Switch{,1..3} (4 alike) : Switch  Criteria=u2 > Threshold
  Terminator : Terminator
  cosδf=1 : Trigonometry  Operator=cos
  cosδr : Trigonometry  Operator=cos
  distribution ratio : Product  Inputs=/*
  f_in : Product
  f_out : Product
  r_in : Product
  r_out : Product
  ratio of f : Product  Inputs=/*
  ratio of f_in : Sum  Inputs=+-
  ratio of f_out : Product  Inputs=/*
  ratio of r : Product  Inputs=/*
  ratio of r_in : Sum  Inputs=+-
  ratio of r_out : Product  Inputs=/*
  sinδf=0 : Trigonometry
  sinδr : Trigonometry
  x_f=0 : Product
  x_r=L : Sum  Inputs=-+
  y_R=R_f : Product
  y_in : Sum  Inputs=+-
  y_out : Sum
  β : Sum  Inputs=+-
  motion_f : Outport
  motion_r : Outport  Port=2
  motion_f_l : Outport  Port=3
  motion_f_r : Outport  Port=4
  motion_r_l : Outport  Port=5
  motion_r_r : Outport  Port=6
  wires:
  L/1 -> R_r'/2, L_r/1, x_r=L/2
  L_f/1 -> L_r/2
  Abs/1 -> sinδf=0/1, cosδf=1/1
  Abs1/1 -> cosδr/1, sinδr/1
  sinδr/1 -> R_r'/1
  cosδf=1/1 -> R_r/1, y_R=R_f/1
  cosδr/1 -> R_f/1
  R_r'/1 -> R_r/2, R_f/2
  R_f/1 -> distribution ratio/2, y_R=R_f/2, x_f=0/2
  R_r/1 -> distribution ratio/1
  distribution ratio/1 -> Add3/1, Divide1/1
  Constant/1 -> ratio of f/2, ratio of r/2, Add2/2, Add3/2, Divide1/2
  Divide1/1 -> Add2/1
  Add2/1 -> ratio of f/1
  Add3/1 -> ratio of r/1
  motion_dem/1 -> Product/2, Product1/1, MATLAB Function/5(motion_dem)
  ratio of r/1 -> Product1/2
  ratio of f/1 -> Product/1
  Product1/1 -> r_out/1, r_in/1, Gain4/1
  Product/1 -> f_in/1, f_out/1, Gain3/1
  β/1 -> Switch3/2, Switch1/2, Switch/2, Switch2/2
  Gain/1 -> Abs/1
  steering angle_r/1 -> β/2, Gain1/1
  Gain1/1 -> Abs1/1
  B/1 -> Gain2/1
  y_R=R_f/1 -> y_out/1, y_in/1
  Gain2/1 -> y_out/2, y_in/2
  sinδf=0/1 -> x_f=0/1
  L_r/1 -> Terminator/1
  x_f=0/1 -> x_r=L/1, Math Function2/1
  y_in/1 -> Math Function/1
  y_out/1 -> Math Function1/1
  x_r=L/1 -> Math Function3/1
  Math Function/1 -> R_r_in^2/1, R_f_in^2/1
  Math Function2/1 -> R_f_out^2/2, R_f_in^2/2
  Math Function1/1 -> R_r_out^2/1, R_f_out^2/1
  Math Function3/1 -> R_r_out^2/2, R_r_in^2/2
  R_f_in^2/1 -> R_f_in/1
  R_r_in^2/1 -> R_r_in/1
  R_f_out^2/1 -> R_f_out/1
  R_r_out^2/1 -> R_r_out/1
  R_f_in/1 -> R_f_tot/1
  R_f_out/1 -> ratio of f_out/2, R_f_tot/2
  R_r_in/1 -> R_r_tot/1
  R_r_out/1 -> ratio of r_out/2, R_r_tot/2
  R_f_tot/1 -> ratio of f_out/1
  R_r_tot/1 -> ratio of r_out/1
  ratio of f_out/1 -> f_out/2, ratio of f_in/2
  ratio of r_out/1 -> r_out/2, ratio of r_in/2
  Constant1/1 -> ratio of f_in/1, ratio of r_in/1
  ratio of r_in/1 -> r_in/2
  ratio of f_in/1 -> f_in/2
  f_in/1 -> Switch1/3, Switch/1
  r_in/1 -> Switch2/1, Switch3/3
  f_out/1 -> Switch/3, Switch1/1
  r_out/1 -> Switch2/3, Switch3/1
  steering angle_f/1 -> Gain/1, β/1
  Gain3/1 -> motion_f/1
  Gain4/1 -> motion_r/1
  Switch/1 -> MATLAB Function/1(fl)
  Switch1/1 -> MATLAB Function/2(fr)
  Switch2/1 -> MATLAB Function/3(rl)
  Switch3/1 -> MATLAB Function/4(rr)
  MATLAB Function/1(motion_fl) -> motion_f_l/1
  MATLAB Function/2(motion_fr) -> motion_f_r/1
  MATLAB Function/3(motion_rl) -> motion_r_l/1
  MATLAB Function/4(motion_rr) -> motion_r_r/1

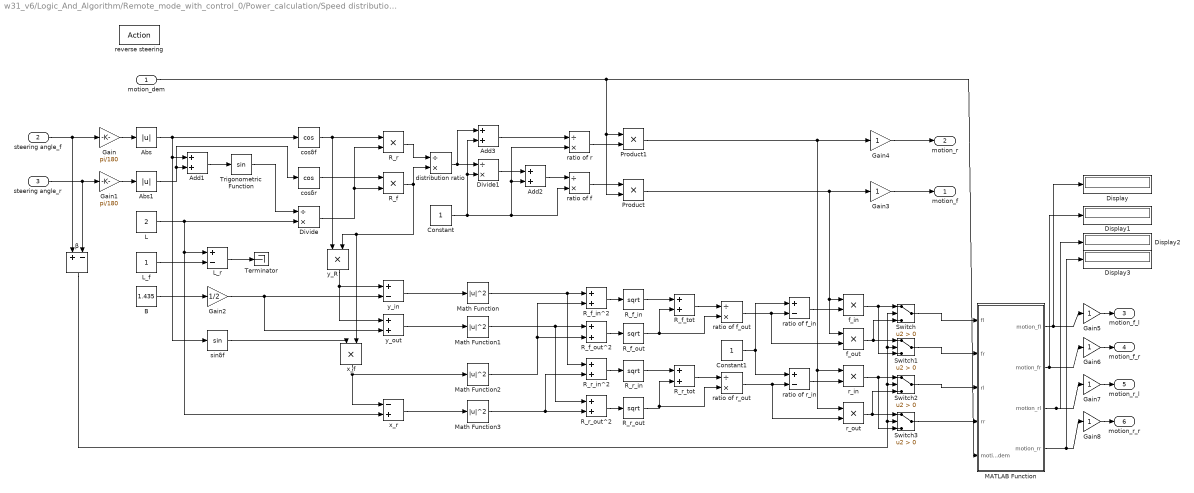
== system w31_v6/Logic_And_Algorithm/Remote_mode_with_control_0/Power_calculation/Speed distribution strategy/motion distribution1/reverse steering ==
  motion_dem : Inport
  steering angle_f : Inport  Port=2
  steering angle_r : Inport  Port=3
  reverse steering : ActionPort  ActionType=case
  Abs : Abs
  Abs1 : Abs
  Add1 : Sum
  Add2 : Sum
  Add3 : Sum
  B : Constant  Value=1.435
  Constant : Constant
  Constant1 : Constant
  Display{,1..3} (4 alike) : Display
  Divide : Product  Inputs=/*
  Divide1 : Product  Inputs=/*
  Gain : Gain  Gain=pi/180
  Gain1 : Gain  Gain=pi/180
  Gain2 : Gain  Gain=1/2
  Gain{3..8} (6 alike) : Gain
  L : Constant  Value=2
  L_f : Constant
  L_r : Sum  Inputs=+-
  MATLAB Function : MATLAB Function  TreatAsAtomicUnit=on
  Math Function{,1..3} (4 alike) : Math  Operator=magnitude^2  SaturateOnIntegerOverflow=on
  Product : Product
  Product1 : Product
  R_f : Product
  R_f_in : Sqrt  SaturateOnIntegerOverflow=on
  R_f_in^2 : Sum
  R_f_out : Sqrt  SaturateOnIntegerOverflow=on
  R_f_out^2 : Sum
  R_f_tot : Sum
  R_r : Product
  R_r_in : Sqrt  SaturateOnIntegerOverflow=on
  R_r_in^2 : Sum
  R_r_out : Sqrt  SaturateOnIntegerOverflow=on
  R_r_out^2 : Sum
  R_r_tot : Sum
  Switch{,1..3} (4 alike) : Switch  Criteria=u2 > Threshold
  Terminator : Terminator
  Trigonometric Function : Trigonometry
  cosδf : Trigonometry  Operator=cos
  cosδr : Trigonometry  Operator=cos
  distribution ratio : Product  Inputs=/*
  f_in : Product
  f_out : Product
  r_in : Product
  r_out : Product
  ratio of f : Product  Inputs=/*
  ratio of f_in : Sum  Inputs=+-
  ratio of f_out : Product  Inputs=/*
  ratio of r : Product  Inputs=/*
  ratio of r_in : Sum  Inputs=+-
  ratio of r_out : Product  Inputs=/*
  sinδf : Trigonometry
  x_f : Product
  x_r : Sum  Inputs=-+
  y_R : Product
  y_in : Sum  Inputs=+-
  y_out : Sum
  β : Sum  Inputs=+-
  motion_f : Outport
  motion_r : Outport  Port=2
  motion_f_l : Outport  Port=3
  motion_f_r : Outport  Port=4
  motion_r_l : Outport  Port=5
  motion_r_r : Outport  Port=6
  wires:
  L/1 -> Divide/2, L_r/1, x_r/2
  L_f/1 -> L_r/2
  Abs/1 -> sinδf/1, Add1/1, cosδf/1
  Abs1/1 -> cosδr/1, Add1/2
  Add1/1 -> Trigonometric Function/1
  Trigonometric Function/1 -> Divide/1
  cosδf/1 -> R_r/1, y_R/1
  cosδr/1 -> R_f/1
  Divide/1 -> R_f/2, R_r/2
  R_f/1 -> y_R/2, x_f/2, distribution ratio/2
  R_r/1 -> distribution ratio/1
  distribution ratio/1 -> Add3/1, Divide1/1
  Constant/1 -> ratio of f/2, ratio of r/2, Add2/2, Add3/2, Divide1/2
  Divide1/1 -> Add2/1
  Add2/1 -> ratio of f/1
  Add3/1 -> ratio of r/1
  motion_dem/1 -> Product/2, Product1/1, MATLAB Function/5(motion_dem)
  ratio of r/1 -> Product1/2
  ratio of f/1 -> Product/1
  Product1/1 -> r_out/1, r_in/1, Gain4/1
  Product/1 -> f_in/1, f_out/1, Gain3/1
  β/1 -> Switch3/2, Switch1/2, Switch/2, Switch2/2
  Gain/1 -> Abs/1
  steering angle_r/1 -> Gain1/1, β/2
  Gain1/1 -> Abs1/1
  B/1 -> Gain2/1
  y_R/1 -> y_out/1, y_in/1
  Gain2/1 -> y_out/2, y_in/2
  sinδf/1 -> x_f/1
  L_r/1 -> Terminator/1
  x_f/1 -> x_r/1, Math Function2/1
  y_in/1 -> Math Function/1
  y_out/1 -> Math Function1/1
  x_r/1 -> Math Function3/1
  Math Function/1 -> R_r_in^2/1, R_f_in^2/1
  Math Function2/1 -> R_f_out^2/2, R_f_in^2/2
  Math Function1/1 -> R_r_out^2/1, R_f_out^2/1
  Math Function3/1 -> R_r_out^2/2, R_r_in^2/2
  R_f_in^2/1 -> R_f_in/1
  R_r_in^2/1 -> R_r_in/1
  R_f_out^2/1 -> R_f_out/1
  R_r_out^2/1 -> R_r_out/1
  R_f_in/1 -> R_f_tot/1
  R_f_out/1 -> ratio of f_out/2, R_f_tot/2
  R_r_in/1 -> R_r_tot/1
  R_r_out/1 -> R_r_tot/2, ratio of r_out/2
  R_f_tot/1 -> ratio of f_out/1
  R_r_tot/1 -> ratio of r_out/1
  ratio of f_out/1 -> f_out/2, ratio of f_in/2
  ratio of r_out/1 -> r_out/2, ratio of r_in/2
  Constant1/1 -> ratio of f_in/1, ratio of r_in/1
  ratio of r_in/1 -> r_in/2
  ratio of f_in/1 -> f_in/2
  f_in/1 -> Switch1/3, Switch/1
  r_in/1 -> Switch2/1, Switch3/3
  f_out/1 -> Switch/3, Switch1/1
  r_out/1 -> Switch2/3, Switch3/1
  steering angle_f/1 -> β/1, Gain/1
  Gain3/1 -> motion_f/1
  Gain4/1 -> motion_r/1
  MATLAB Function/1(motion_fl) -> Gain5/1, Display/1
  MATLAB Function/2(motion_fr) -> Gain6/1, Display1/1
  MATLAB Function/3(motion_rl) -> Gain7/1, Display2/1
  MATLAB Function/4(motion_rr) -> Gain8/1, Display3/1
  Switch/1 -> MATLAB Function/1(fl)
  Switch1/1 -> MATLAB Function/2(fr)
  Switch2/1 -> MATLAB Function/3(rl)
  Switch3/1 -> MATLAB Function/4(rr)
  Gain5/1 -> motion_f_l/1
  Gain6/1 -> motion_f_r/1
  Gain7/1 -> motion_r_l/1
  Gain8/1 -> motion_r_r/1

== system w31_v6/Logic_And_Algorithm/iECU_mode_with_control/Power_calculation/PID_Controller/FL_PI_Cal2/PI ==
  Error : Inport
  PID_Reset : Inport  Port=2
  Igain : Inport  Port=3
  Pgain : Inport  Port=4
  Clamping circuit : Subsystem
  Constant : Constant  Value=0
  Discrete-Time Integrator : DiscreteIntegrator  ExternalReset=level  InitialConditionMode=State only (most efficient)  SampleTime=-1  ICPrevOutput=DiscIntNeverNeededParam  ICPrevScaledInput=DiscIntNeverNeededParam
  Product : Product  RndMeth=Zero
  Product1 : Product  RndMeth=Zero
  Saturation : Saturate  UpperLimit=300  LowerLimit=0
  Sum : Sum  Inputs=++|
  Switch : Switch  Criteria=u2 > Threshold
  PI_闭环计算扭矩 : Outport
  wires:
  Pgain/1 -> Product1/1
  Igain/1 -> Product/2
  Product1/1 -> Sum/1
  PID_Reset/1 -> Discrete-Time Integrator/2
  Saturation/1 -> PI_闭环计算扭矩/1
  Sum/1 -> Clamping circuit/1(preSat), Saturation/1
  Discrete-Time Integrator/1 -> Sum/2
  Switch/1 -> Discrete-Time Integrator/1
  Clamping circuit/1(Clamp) -> Switch/2
  Product/1 -> Clamping circuit/2(preIntegrator), Switch/3
  Constant/1 -> Switch/1
  Error/1 -> Product1/2, Product/1

== system w31_v6/Logic_And_Algorithm/iECU_mode_with_control/Power_calculation/PID_Controller/FR_PI_Cal1/PI ==
  Error : Inport
  PID_Reset : Inport  Port=2
  Igain : Inport  Port=3
  Pgain : Inport  Port=4
  Clamping circuit : Subsystem
  Constant : Constant  Value=0
  Discrete-Time Integrator : DiscreteIntegrator  ExternalReset=level  InitialConditionMode=State only (most efficient)  SampleTime=-1  ICPrevOutput=DiscIntNeverNeededParam  ICPrevScaledInput=DiscIntNeverNeededParam
  Product : Product  RndMeth=Zero
  Product1 : Product  RndMeth=Zero
  Saturation : Saturate  UpperLimit=300  LowerLimit=0
  Sum : Sum  Inputs=++|
  Switch : Switch  Criteria=u2 > Threshold
  PI_闭环计算扭矩 : Outport
  wires:
  Error/1 -> Product/1, Product1/2
  Constant/1 -> Switch/1
  Product/1 -> Switch/3, Clamping circuit/2(preIntegrator)
  Clamping circuit/1(Clamp) -> Switch/2
  Switch/1 -> Discrete-Time Integrator/1
  Discrete-Time Integrator/1 -> Sum/2
  Sum/1 -> Saturation/1, Clamping circuit/1(preSat)
  Saturation/1 -> PI_闭环计算扭矩/1
  PID_Reset/1 -> Discrete-Time Integrator/2
  Product1/1 -> Sum/1
  Igain/1 -> Product/2
  Pgain/1 -> Product1/1

== system w31_v6/Logic_And_Algorithm/iECU_mode_with_control/Power_calculation/PID_Controller/RL_PI_Cal/PI ==
  Error : Inport
  PID_Reset : Inport  Port=2
  Igain : Inport  Port=3
  Pgain : Inport  Port=4
  Clamping circuit : Subsystem
  Constant : Constant  Value=0
  Discrete-Time Integrator : DiscreteIntegrator  ExternalReset=level  InitialConditionMode=State only (most efficient)  SampleTime=-1  ICPrevOutput=DiscIntNeverNeededParam  ICPrevScaledInput=DiscIntNeverNeededParam
  Product : Product  RndMeth=Zero
  Product1 : Product  RndMeth=Zero
  Saturation : Saturate  UpperLimit=300  LowerLimit=0
  Sum : Sum  Inputs=++|
  Switch : Switch  Criteria=u2 > Threshold
  PI_闭环计算扭矩 : Outport
  wires:
  Error/1 -> Product/1, Product1/2
  Constant/1 -> Switch/1
  Product/1 -> Switch/3, Clamping circuit/2(preIntegrator)
  Clamping circuit/1(Clamp) -> Switch/2
  Switch/1 -> Discrete-Time Integrator/1
  Discrete-Time Integrator/1 -> Sum/2
  Sum/1 -> Saturation/1, Clamping circuit/1(preSat)
  Saturation/1 -> PI_闭环计算扭矩/1
  PID_Reset/1 -> Discrete-Time Integrator/2
  Product1/1 -> Sum/1
  Igain/1 -> Product/2
  Pgain/1 -> Product1/1

== system w31_v6/Logic_And_Algorithm/iECU_mode_with_control/Power_calculation/PID_Controller/RR_PI_Cal/PI ==
  Error : Inport
  PID_Reset : Inport  Port=2
  Igain : Inport  Port=3
  Pgain : Inport  Port=4
  Clamping circuit : Subsystem
  Constant : Constant  Value=0
  Discrete-Time Integrator : DiscreteIntegrator  ExternalReset=level  InitialConditionMode=State only (most efficient)  SampleTime=-1  ICPrevOutput=DiscIntNeverNeededParam  ICPrevScaledInput=DiscIntNeverNeededParam
  Product : Product  RndMeth=Zero
  Product1 : Product  RndMeth=Zero
  Saturation : Saturate  UpperLimit=300  LowerLimit=0
  Sum : Sum  Inputs=++|
  Switch : Switch  Criteria=u2 > Threshold
  PI_闭环计算扭矩 : Outport
  wires:
  Error/1 -> Product/1, Product1/2
  Constant/1 -> Switch/1
  Product/1 -> Switch/3, Clamping circuit/2(preIntegrator)
  Clamping circuit/1(Clamp) -> Switch/2
  Switch/1 -> Discrete-Time Integrator/1
  Discrete-Time Integrator/1 -> Sum/2
  Sum/1 -> Saturation/1, Clamping circuit/1(preSat)
  Saturation/1 -> PI_闭环计算扭矩/1
  PID_Reset/1 -> Discrete-Time Integrator/2
  Product1/1 -> Sum/1
  Igain/1 -> Product/2
  Pgain/1 -> Product1/1

== system w31_v6/Logic_And_Algorithm/iECU_mode_with_control/Power_calculation/PID_Controller/FL_PI_Cal2/PI/Clamping circuit ==
  preSat : Inport
  preIntegrator : Inport  Port=2
  Data Type Conversion : DataTypeConversion  OutDataTypeStr=int8  RndMeth=Zero
  Data Type Conversion1 : DataTypeConversion  OutDataTypeStr=int8
  Dead Zone : DeadZone  LowerValue=-250  UpperValue=250
  Logical Operator : Logic  AllPortsSameDT=off  OutDataTypeStr=boolean
  Relational Operator : RelationalOperator  Operator=~=
  Relational Operator1 : RelationalOperator  Operator===
  Sign : Signum
  Sign1 : Signum
  ZeroGain : Gain  Gain=0
  Clamp : Outport
  wires:
  Logical Operator/1 -> Clamp/1
  Relational Operator1/1 -> Logical Operator/2
  Relational Operator/1 -> Logical Operator/1
  Data Type Conversion1/1 -> Relational Operator1/2
  Sign1/1 -> Data Type Conversion1/1
  preIntegrator/1 -> Sign1/1
  Data Type Conversion/1 -> Relational Operator1/1
  Sign/1 -> Data Type Conversion/1
  Dead Zone/1 -> Relational Operator/2, Sign/1
  ZeroGain/1 -> Relational Operator/1
  preSat/1 -> Dead Zone/1, ZeroGain/1

== system w31_v6/Logic_And_Algorithm/iECU_mode_with_control/Power_calculation/PID_Controller/FR_PI_Cal1/PI/Clamping circuit ==
  preSat : Inport
  preIntegrator : Inport  Port=2
  Data Type Conversion : DataTypeConversion  OutDataTypeStr=int8  RndMeth=Zero
  Data Type Conversion1 : DataTypeConversion  OutDataTypeStr=int8
  Dead Zone : DeadZone  LowerValue=-250  UpperValue=250
  Logical Operator : Logic  AllPortsSameDT=off  OutDataTypeStr=boolean
  Relational Operator : RelationalOperator  Operator=~=
  Relational Operator1 : RelationalOperator  Operator===
  Sign : Signum
  Sign1 : Signum
  ZeroGain : Gain  Gain=0
  Clamp : Outport
  wires:
  preSat/1 -> ZeroGain/1, Dead Zone/1
  ZeroGain/1 -> Relational Operator/1
  Dead Zone/1 -> Sign/1, Relational Operator/2
  Sign/1 -> Data Type Conversion/1
  Data Type Conversion/1 -> Relational Operator1/1
  preIntegrator/1 -> Sign1/1
  Sign1/1 -> Data Type Conversion1/1
  Data Type Conversion1/1 -> Relational Operator1/2
  Relational Operator/1 -> Logical Operator/1
  Relational Operator1/1 -> Logical Operator/2
  Logical Operator/1 -> Clamp/1

== system w31_v6/Logic_And_Algorithm/iECU_mode_with_control/Power_calculation/PID_Controller/RL_PI_Cal/PI/Clamping circuit ==
  preSat : Inport
  preIntegrator : Inport  Port=2
  Data Type Conversion : DataTypeConversion  OutDataTypeStr=int8  RndMeth=Zero
  Data Type Conversion1 : DataTypeConversion  OutDataTypeStr=int8
  Dead Zone : DeadZone  LowerValue=-250  UpperValue=250
  Logical Operator : Logic  AllPortsSameDT=off  OutDataTypeStr=boolean
  Relational Operator : RelationalOperator  Operator=~=
  Relational Operator1 : RelationalOperator  Operator===
  Sign : Signum
  Sign1 : Signum
  ZeroGain : Gain  Gain=0
  Clamp : Outport
  wires:
  preSat/1 -> ZeroGain/1, Dead Zone/1
  ZeroGain/1 -> Relational Operator/1
  Dead Zone/1 -> Sign/1, Relational Operator/2
  Sign/1 -> Data Type Conversion/1
  Data Type Conversion/1 -> Relational Operator1/1
  preIntegrator/1 -> Sign1/1
  Sign1/1 -> Data Type Conversion1/1
  Data Type Conversion1/1 -> Relational Operator1/2
  Relational Operator/1 -> Logical Operator/1
  Relational Operator1/1 -> Logical Operator/2
  Logical Operator/1 -> Clamp/1

== system w31_v6/Logic_And_Algorithm/iECU_mode_with_control/Power_calculation/PID_Controller/RR_PI_Cal/PI/Clamping circuit ==
  preSat : Inport
  preIntegrator : Inport  Port=2
  Data Type Conversion : DataTypeConversion  OutDataTypeStr=int8  RndMeth=Zero
  Data Type Conversion1 : DataTypeConversion  OutDataTypeStr=int8
  Dead Zone : DeadZone  LowerValue=-250  UpperValue=250
  Logical Operator : Logic  AllPortsSameDT=off  OutDataTypeStr=boolean
  Relational Operator : RelationalOperator  Operator=~=
  Relational Operator1 : RelationalOperator  Operator===
  Sign : Signum
  Sign1 : Signum
  ZeroGain : Gain  Gain=0
  Clamp : Outport
  wires:
  preSat/1 -> ZeroGain/1, Dead Zone/1
  ZeroGain/1 -> Relational Operator/1
  Dead Zone/1 -> Sign/1, Relational Operator/2
  Sign/1 -> Data Type Conversion/1
  Data Type Conversion/1 -> Relational Operator1/1
  preIntegrator/1 -> Sign1/1
  Sign1/1 -> Data Type Conversion1/1
  Data Type Conversion1/1 -> Relational Operator1/2
  Relational Operator/1 -> Logical Operator/1
  Relational Operator1/1 -> Logical Operator/2
  Logical Operator/1 -> Clamp/1

== stateflow chart CAN_Receive_10ms/Chassis_CAN/FL_Motor_NoMsg/Chart ==
  state MsgNotRecieve
    en:
    NoRxMsgComfirm=0;
    du:
    NoRxMsgCnt++;
  state MsgRecieve
    en:
    NoRxMsgCnt=0;
    NoRxMsgComfirm=0;
  state MsgNotRecieveComfirm
    en:
    NoRxMsgComfirm=1;
    du:
    NoRxMsgCnt++;
  note: NoRxMsgCnt在RxMsg==0的情况下（CAN信息没有在规定的周期内及时更新）
      | 一直往上加，直到RxMsg==1，NoRxMsgCnt清零。（程序接收到新的CAN信息）。NoRxMsgCnt只受到RxMsg控制。
  note: NoRxMsgComfirm受NoRxMsgCnt和NoRxMsgCntMax两个量控制
      | NoRxmsgComfirm==1没有接收到消息
  state NoRxMsgCntOverFlow
    en:
    NoRxMsgCnt=65000;
  (default) -> MsgNotRecieve : {NoRxMsgCnt=0;}
  MsgNotRecieve -> MsgRecieve [order 1] : [1==RxMsg]
  NoRxMsgCntOverFlow -> MsgRecieve : [1==RxMsg]
  MsgRecieve -> MsgNotRecieve : [0==RxMsg]
  MsgNotRecieveComfirm -> MsgRecieve [order 1] : [1==RxMsg]
  MsgNotRecieve -> MsgNotRecieveComfirm [order 2] : [NoRxMsgCnt>NoRxMsgCntMax]
  MsgNotRecieveComfirm -> NoRxMsgCntOverFlow [order 2] : [NoRxMsgCnt>=65000]
  data: NoRxMsgComfirm output boolean; RxMsg input boolean; NoRxMsgCnt output single; NoRxMsgCntMax input single

== stateflow chart CAN_Receive_10ms/Chassis_CAN/FR_Motor_NoMsg/Chart ==
  state MsgNotRecieve
    en:
    NoRxMsgComfirm=0;
    du:
    NoRxMsgCnt++;
  state MsgRecieve
    en:
    NoRxMsgCnt=0;
    NoRxMsgComfirm=0;
  state MsgNotRecieveComfirm
    en:
    NoRxMsgComfirm=1;
    du:
    NoRxMsgCnt++;
  note: NoRxMsgCnt在RxMsg==0的情况下（CAN信息没有在规定的周期内及时更新）
      | 一直往上加，直到RxMsg==1，NoRxMsgCnt清零。（程序接收到新的CAN信息）。NoRxMsgCnt只受到RxMsg控制。
  note: NoRxMsgComfirm受NoRxMsgCnt和NoRxMsgCntMax两个量控制
      | NoRxmsgComfirm==1没有接收到消息
  state NoRxMsgCntOverFlow
    en:
    NoRxMsgCnt=65000;
  (default) -> MsgNotRecieve : {NoRxMsgCnt=0;}
  MsgNotRecieve -> MsgRecieve [order 1] : [1==RxMsg]
  NoRxMsgCntOverFlow -> MsgRecieve : [1==RxMsg]
  MsgRecieve -> MsgNotRecieve : [0==RxMsg]
  MsgNotRecieveComfirm -> MsgRecieve [order 1] : [1==RxMsg]
  MsgNotRecieve -> MsgNotRecieveComfirm [order 2] : [NoRxMsgCnt>NoRxMsgCntMax]
  MsgNotRecieveComfirm -> NoRxMsgCntOverFlow [order 2] : [NoRxMsgCnt>=65000]
  data: NoRxMsgComfirm output boolean; RxMsg input boolean; NoRxMsgCnt output single; NoRxMsgCntMax input single

== stateflow chart CAN_Receive_10ms/Remote_Control_CAN/shake_situation1/Chart ==
  state MsgNotRecieve
    en:
    NoRxMsgComfirm=0;
    du:
    NoRxMsgCnt++;
  state MsgRecieve
    en:
    NoRxMsgCnt=0;
    NoRxMsgComfirm=0;
  state MsgNotRecieveComfirm
    en:
    NoRxMsgComfirm=1;
    du:
    NoRxMsgCnt++;
  note: NoRxMsgCnt在RxMsg==0的情况下（CAN信息没有在规定的周期内及时更新）
      | 一直往上加，直到RxMsg==1，NoRxMsgCnt清零。（程序接收到新的CAN信息）。NoRxMsgCnt只受到RxMsg控制。
  note: NoRxMsgComfirm受NoRxMsgCnt和NoRxMsgCntMax两个量控制
      | NoRxmsgComfirm==1没有接收到消息
  state NoRxMsgCntOverFlow
    en:
    NoRxMsgCnt=65000;
  (default) -> MsgNotRecieve : {NoRxMsgCnt=0;}
  MsgNotRecieve -> MsgRecieve [order 1] : [1==RxMsg]
  NoRxMsgCntOverFlow -> MsgRecieve : [1==RxMsg]
  MsgRecieve -> MsgNotRecieve : [0==RxMsg]
  MsgNotRecieveComfirm -> MsgRecieve [order 1] : [1==RxMsg]
  MsgNotRecieve -> MsgNotRecieveComfirm [order 2] : [NoRxMsgCnt>NoRxMsgCntMax]
  MsgNotRecieveComfirm -> NoRxMsgCntOverFlow [order 2] : [NoRxMsgCnt>=65000]
  data: NoRxMsgComfirm output boolean; RxMsg input boolean; NoRxMsgCnt output single; NoRxMsgCntMax input single
